simulink model "psbsurgnetwork"  (Simulink 6.0)
settings: Solver=ode15s  SolverMode=SingleTasking  StartTime=0.0  StopTime=0.2  RelTol=1e-3  AbsTol=1e-2
libraries: powerlib2 x24
settings Model: Creator=patrice  LastModifiedBy=batserve  ExtModeTrigMode=oneshot  ExtModeArmWhenConnect=off  ExtModeAutoUpdateStatusClock=off
settings DataIOCC: LimitDataPoints=off  SignalLoggingName=sigsOut
settings OptimizationCC: BlockReduction=off  BooleanDataType=off
settings DebuggingCC: AlgebraicLoopMsg=none  CheckExecutionContextPreStartOutputMsg=on  CheckExecutionContextRuntimeOutputMsg=on  SolverPrmCheckMsg=none
settings HardwareCC: TargetUnknown=on
settings RTWCC: TemplateMakefile=grt_unix.tmf

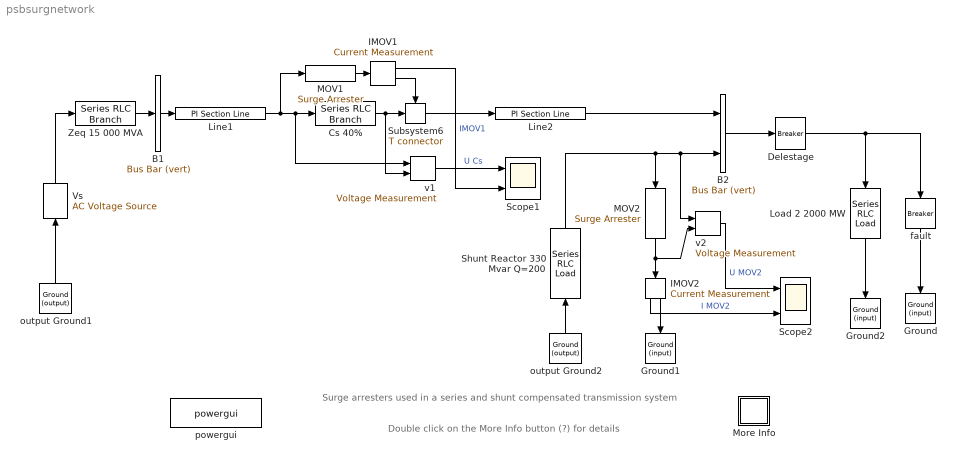
== system psbsurgnetwork ==
  note: Double click on the More Info button (?) for details
  note: Surge arresters used in  a series and shunt  compensated
      |  transmission system
  B1 : powerlib2/Connectors/Bus Bar (vert)  Tag=PoWeRsYsTeMbLoCk  entrees=1  sorties=1  PSBOutputType=11111111111111111111111111111111111111111111111111111111111111111111111111111111111111111
  B2 : powerlib2/Connectors/Bus Bar (vert)  Tag=PoWeRsYsTeMbLoCk  entrees=2  sorties=1  PSBOutputType=11111111111111111111111111111111111111111111111111111111111111111111111111111111111111111
  Cs 40% : powerlib2/Elements/Series RLC Branch  Tag=PoWeRsYsTeMbLoCk  a=0  b=0  c=101.4e-6  mesure=None  PSBOutputType=1
  Delestage : powerlib2/Elements/Breaker  Tag=PoWeRsYsTeMbLoCk  a=0.1  c=1  rs=inf  cs=0  times=[ 100e-3]  Ts=0  comext=off  mesure=None  PSBOutputType=1
  Ground : powerlib2/Connectors/Ground (input)  Tag=PoWeRsYsTeMbLoCk  Orientation=down
  Ground1 : powerlib2/Connectors/Ground (input)  Tag=PoWeRsYsTeMbLoCk  Orientation=down
  Ground2 : powerlib2/Connectors/Ground (input)  Tag=PoWeRsYsTeMbLoCk  Orientation=down
  IMOV1 : powerlib2/Measurements/Current Measurement  Tag=PoWeRsYsTeMmEaSuReMeNt  PhasorSimulation=off  OutputType=Magnitude  PSBOutputType=01  PSBequivalent=0
  IMOV2 : powerlib2/Measurements/Current Measurement  Tag=PoWeRsYsTeMmEaSuReMeNt  Orientation=down  PhasorSimulation=off  OutputType=Magnitude  PSBOutputType=01  PSBequivalent=0
  Line1 : powerlib2/Elements/PI Section Line  Tag=PoWeRsYsTeMbLoCk  f=60  a=0.011  b=0.8674e-3  c=13.41e-9  d=100  e=2  mesure=None  PSBOutputType=1
  Line2 : powerlib2/Elements/PI Section Line  Tag=PoWeRsYsTeMbLoCk  f=60  a=0.011  b=0.8674e-3  c=13.41e-9  d=100  e=2  mesure=None  PSBOutputType=1
  Load 2 2000 MW : powerlib2/Elements/Series RLC Load  Tag=PoWeRsYsTeMbLoCk  Orientation=down  a=735e3/sqrt(3)  b=60  c=2000e6/3  d=0  e=0  mesure=None  PSBOutputType=1
  MOV1 : powerlib2/Elements/Surge Arrester  Tag=PoWeRsYsTeMbLoCk  x1=185e3  x2=30  x3=500  x4=[.955 50]  x5=[1.0 25]  x6=[.9915 16.5]  mesure=None  PSBOutputType=1
  MOV2 : powerlib2/Elements/Surge Arrester  Tag=PoWeRsYsTeMbLoCk  Orientation=down  x1=1081e3  x2=2  x3=500  x4=[.955 50]  x5=[1.0 25]  x6=[.9915 16.5]  mesure=None  PSBOutputType=1
  More Info : Subsystem
      mask Display: disp('?')
  Scope1 : Scope  NumInputPorts=2
      settings: TimeRange=0.2  YMin=-200000~-5000  YMax=200000~10000  DataFormat=Array  MaxDataPoints=500000
  Scope2 : Scope  NumInputPorts=2
      settings: TimeRange=0.2  YMin=-2e+006~0  YMax=2e+006~1000  DataFormat=Array  MaxDataPoints=500000
  Shunt Reactor 330 Mvar Q=200 : powerlib2/Elements/Series RLC Load  Tag=PoWeRsYsTeMbLoCk  Orientation=up  a=735e3/sqrt(3)  b=60  c=330e6/3/200  d=330e6/3  e=0  mesure=None  PSBOutputType=1
  Subsystem6 : powerlib2/Connectors/T connector  Tag=PoWeRsYsTeMbLoCk  PSBOutputType=1
  Vs : powerlib2/Electrical Sources/AC Voltage Source  Tag=PoWeRsYsTeMbLoCk  Orientation=up  A=735e3/sqrt(3)*sqrt(2)  P=0  F=60  stime=0  mesure=None  PSBOutputType=1
  Zeq 15 000 MVA : powerlib2/Elements/Series RLC Branch  Tag=PoWeRsYsTeMbLoCk  a=3.6  b=95.5e-3  c=inf  mesure=None  PSBOutputType=1
  fault : powerlib2/Elements/Breaker  Tag=PoWeRsYsTeMbLoCk  Orientation=down  a=1  c=0  rs=inf  cs=0  times=[ 30e-3 300e-3]  Ts=0  comext=off  mesure=None  PSBOutputType=1
  output Ground1 : powerlib2/Connectors/Ground (output)  Tag=PoWeRsYsTeMbLoCk  Orientation=up  PSBOutputType=1
  output Ground2 : powerlib2/Connectors/Ground (output)  Tag=PoWeRsYsTeMbLoCk  Orientation=up  PSBOutputType=1
  powergui : powerlib2/powergui  Frange=logspace(0,3,50)  Ylog=off  Xlog=off  save=off  variable=ZData  ZoomFFT=on  StartTime=0.0  cycles=1  DisplayStyle=off  fundamental=60  FreqAxis=off  MaxFrequency=1000  frequencyindice=1  frequencyindicesteady=1  RmsSteady=1  display=off  Ts=0  methode=off  frequency=60  echomessages=off
  v1 : powerlib2/Measurements/Voltage Measurement  Tag=PoWeRsYsTeMmEaSuReMeNt  PhasorSimulation=off  OutputType=Magnitude  PSBOutputType=0  PSBequivalent=0
  v2 : powerlib2/Measurements/Voltage Measurement  Tag=PoWeRsYsTeMmEaSuReMeNt  PhasorSimulation=off  OutputType=Magnitude  PSBOutputType=0  PSBequivalent=0
  wires:
  output Ground1/1 -> Vs/1
  Vs/1 -> Zeq 15 000 MVA/1
  v2/1 -> Scope2/1  "U MOV2"
  Line2/1 -> B2/1
  B2/1 -> Delestage/1
  Zeq 15 000 MVA/1 -> B1/1
  B1/1 -> Line1/1
  MOV1/1 -> IMOV1/1
  Line1/1 -> MOV1/1, Cs 40%/1, v1/1
  IMOV1/2 -> Subsystem6/Enable
  Subsystem6/1 -> Line2/1
  Cs 40%/1 -> Subsystem6/1, v1/2
  Shunt Reactor 330 Mvar Q=200/1 -> B2/2, v2/1, MOV2/1
  output Ground2/1 -> Shunt Reactor 330 Mvar Q=200/1
  IMOV2/1 -> Scope2/2  "I MOV2"
  fault/1 -> Ground/1
  Load 2 2000 MW/1 -> Ground2/1
  Delestage/1 -> Load 2 2000 MW/1, fault/1
  v1/1 -> Scope1/1  "U Cs"
  IMOV1/1 -> Scope1/2  "IMOV1"
  MOV2/1 -> IMOV2/1, v2/2
  IMOV2/2 -> Ground1/1

== system psbsurgnetwork/More Info ==
  note: Start the simulation.  Observe the MOV voltages and currents on Scope1 and Scope2.
      |
      | At fault application  the capacitor voltage increases and  MOV1 conducts. Peak current  reaches  8.4 kA on the 2nd pulse
      | 2 cycles after fault application,  the MOV current is symetric  (4.5 kA current pulses at every half cycle).
      |
      | At fault clearing, the  overvoltage  produced at bus B2 is limited by the shunt MOV2 .
      | The fast transient produces a 850 A current pulse in the MOV.
  note: A 735 kV equivalent transmission systems feeds a load through a 200 km transmission line. The line is series compensated at the
      | middle point and shunt compensated at its receiving end.  A fault  is applied at the load terminals.
      | The fault is cleared by load breaker opening. For simplification purpose, only  one phase of the transmission system is modelled.
      | All parameters correspond to positive-sequence.
      |
      | The  three-phase  short circuit level of the transmission system is 15000 MVA. The line is 40% series compensated by a capacitor
      | (26.2 ohms at 60 Hz) and shunt compensated by a 330 Mvar (110 Mvar/phase) inductor  at the load end.
      |
      | The series capacitor and shunt inductor are both protected by metal oxide varistors (MOV).
      | The series capacitor  varistor  MOV1 consists of 30 columns protecting the capacitor at 2.5 times
      | its rated voltage (rated voltage is obtained for a 2000 kA line rated current).
      | The corresponding protection  voltage (defined at 15 kA =  500 A per column)  is  2.5*26.2 *2kA*sqrt(2)=185 kV.
      |
      | The shunt inductor is protected by a 2-column arrester  (MOV2) at 1.8 p.u. of nominal
      | phase-to-ground voltage (424.4 kVrms). The corresponding protection voltage (defined at 1 kA or 500A /column)
      | is 1.8*424.4*sqrt(2)= 1080 kV.
  note: This demonstration illustrates use of surge arresters in a
      | series and shunt compensated 735 kV AC transmission system
  note: Circuit Description
  note: Demonstration
  note: G. Sybille (Hydro-Quebec)
